simulink library "GearSystems"  (R2023b)
settings: Solver=VariableStepAuto  StartTime=0.0  StopTime=10.0  RelTol=1e-3
undefined symbols (not defined in the file or in its folder): manual_gearbox
settings Model: Creator=dadikozyanaa  LastModifiedBy=koenjacobs
settings DebuggingCC: UnconnectedInputMsg=warning  UnconnectedOutputMsg=warning  UnconnectedLineMsg=warning
settings ModelReferenceCC: EnableRefExpFcnMdlSchedulingChecks=on
settings RTWCC: DLArmComputeVersion=19.05

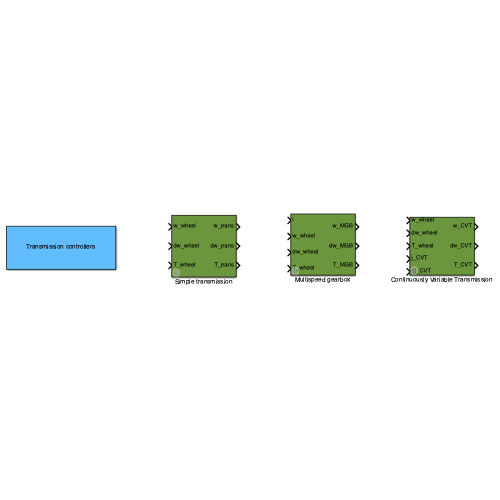
[thumbnail: Simulink's stored preview of the top-level diagram]
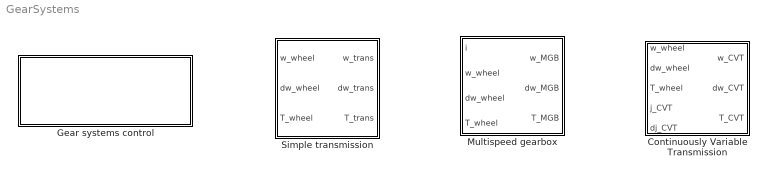
== system GearSystems ==
  Continuously Variable Transmission : Subsystem  Tag=cvt  mask(CVT){e_CVT=0.96, w_max=100, w_wheel_min=1}
      mask prompts: e_CVT "Efficiency [-]"; w_max "Maximum engine speed [rad/s]"; w_wheel_min "Minimum wheel speed beyond which losses are generated [rad/s]"
      mask help:
      | This block simulates a CVT transmission.
      |
      | Input:
      | =====
      | 	w_wheel	Speed of the wheel [rad/s]
      | 	dw_wheel	Acceleration of the wheel [rad/s^2],
      | 	T_wheel	Torque on the wheel [Nm]
      | 	j_CVT	Gear ratio [-]
      | 	dj_CVT	Change of gear ratio [1/s]
      |
      | Output:
      | ======
      | 	w_CVT	Speed of the fly wheel [rad/s]
      | 	dw_CVT	Acceleration of the fly wheel [rad/s^2]
      | 	T_CVT	Torque on the fly wheel [Nm]
      mask init:
      | init_CVT;
  Gear systems control : Subsystem
      settings: OpenFcn=GearSystemsControl
      mask Display:
      | disp(['Transmission controllers' ...
      |     ''])
  Multispeed gearbox : Subsystem  Tag=transmission  mask(Manual Gear Box){nr_gears=2, i_1=15.174, i_2=8.338, i_3=5.378, i_4=3.937, i_5=2.748, i_6=2.748, i_diff=1, e_GT=0.98, P_GT0=300, w_wheel_min=1}
      mask prompts: nr_gears "Select number of gears:"; i_1 "1. gear [-]"; i_2 "2. gear [-]"; i_3 "3. gear [-]"; i_4 "4. gear [-]"; i_5 "5. gear [-]"; i_6 "6. gear [-]"; i_diff "Differential gear [-]"; e_GT "Efficiency [-]"; P_GT0 "Idling losses (friction) [W]"; w_wheel_min "Minimum wheel speed beyond which losses are generated [rad/s]"
      mask help:
      | This block simulates a manual gear box.
      |
      | Input:
      | =====
      | 	w_wheel	Speed of the wheel [rad/s]
      | 	dw_wheel	Acceleration of the wheel [rad/s^2],
      | 	T_wheel	Torque on the wheel [Nm]
      | 	i	Gear number [-]
      |
      | Output:
      | ======
      | 	w_MGB	Speed of the fly wheel [rad/s]
      | 	dw_MGB	Acceleration of the fly wheel [rad/s^2]
      | 	T_MGB	Torque on the fly wheel [Nm]
      mask init:
      | init_MGB;
      | init_MGB_control;
      mask Help: Contact a.a.dadikozyan@student.tue.nl for help.
      mask TypeOptions nr_gears: 2 | 3 | 4 | 5 | 6
      mask Callback nr_gears:
      | maskStr = get_param(gcb,'nr_gears');
      | 
      | switch maskStr
      |     case '2'
      |         set_param(gcb,'MaskVisibilities',{'on';'on';'on';'off';'off';'off';'off';'on';'on';'on';'on'}),
      |     case '3'
      |         set_param(gcb,'MaskVisibilities',{'on';'on';'on';'on';'off';'off';'off';'on';'on';'on';'on'}),
      |     case '4'
      |         set_param(gcb,'MaskVisibilities',{'on';'on';'on';'on';'on';'off';'off';'on';'on';'on';'on'}),
      |     case '5'
      |         set_param(gcb,'MaskVisibilities',{'on';'on';'on';'on';'on';'on';'off';'on';'on';'on';'on'}),
      |     case '6'
      |         set_param(gcb,'MaskVisibilities',{'on';'on';'on';'on';'on';'on';'on';'on';'on';'on';'on'}),
      | end
      | 
      | %set_param(gcb,'editvalue',maskStr);
  Simple transmission : Subsystem  mask(Simple Transmission){gear_ratio=3, e_GT=0.98, P_GT0=50, w_wheel_min=1}
      mask prompts: gear_ratio "Gear ratio [-]"; e_GT "Efficiency [-]"; P_GT0 "Idling losses (friction) [W]"; w_wheel_min "Minimum wheel speed beyond which losses are generated [rad/s]"
      mask help:
      | This block simulates a transmission with a fixed gear ratio.
      |
      | Input:
      | =====
      | 	w_wheel	Speed of the wheel [rad/s]
      | 	dw_wheel	Acceleration of the wheel [rad/s^2]
      | 	T_wheel	Torque on the wheel [Nm]
      |
      | Output:
      | ======
      | 	w_trans	Speed of the fly wheel [rad/s]
      | 	dw_trans	Acceleration of the fly wheel [rad/s^2]
      | 	T_trans	Torque on the fly wheel [Nm]
      mask init:
      | init_transmission

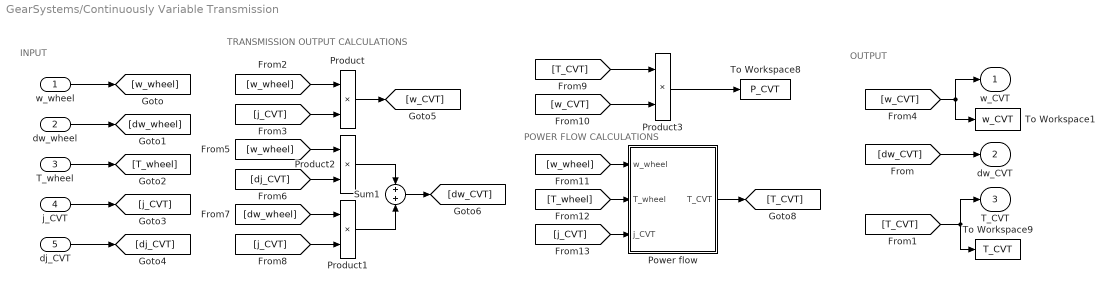
== system GearSystems/Continuously Variable Transmission ==
  note: POWER FLOW CALCULATIONS
  note: TRANSMISSION OUTPUT CALCULATIONS
  note: OUTPUT
  note: INPUT
  w_wheel : Inport
  dw_wheel : Inport  Port=2
  T_wheel : Inport  Port=3
  j_CVT : Inport  Port=4
  dj_CVT : Inport  Port=5
  Power flow : Subsystem
  Product{,1..3} (4 alike) : Product  InputSameDT=on  RndMeth=Zero  SaturateOnIntegerOverflow=on  OutDataTypeStr=Inherit: Same as first input
  Sum1 : Sum  Inputs=+|+
  To Workspace1 : ToWorkspace  VariableName=w_CVT  SampleTime=-1
  To Workspace8 : ToWorkspace  VariableName=P_CVT  SampleTime=-1
  To Workspace9 : ToWorkspace  VariableName=T_CVT  SampleTime=-1
  w_CVT : Outport  InitialOutput=0
  dw_CVT : Outport  Port=2  InitialOutput=0
  T_CVT : Outport  Port=3  InitialOutput=0
  wires:
  Product1/1 -> Sum1/2
  Product2/1 -> Sum1/1
  w_wheel/1 -> [w_wheel]
  dw_wheel/1 -> [dw_wheel]
  T_wheel/1 -> [T_wheel]
  j_CVT/1 -> [j_CVT]
  dj_CVT/1 -> [dj_CVT]
  [j_CVT] -> Product/2
  [w_wheel] -> Product/1
  [w_wheel] -> Product2/1
  [j_CVT] -> Product1/2
  [dj_CVT] -> Product2/2
  [dw_wheel] -> Product1/1
  Product/1 -> [w_CVT]
  Sum1/1 -> [dw_CVT]
  [w_CVT] -> Product3/2
  [T_CVT] -> Product3/1
  Product3/1 -> To Workspace8/1
  Power flow/1(T_CVT) -> [T_CVT]
  [w_wheel] -> Power flow/1(w_wheel)
  [T_wheel] -> Power flow/2(T_wheel)
  [j_CVT] -> Power flow/3(j_CVT)
  [w_CVT] -> To Workspace1/1, w_CVT/1
  [dw_CVT] -> dw_CVT/1
  [T_CVT] -> To Workspace9/1, T_CVT/1

== system GearSystems/Gear systems control ==

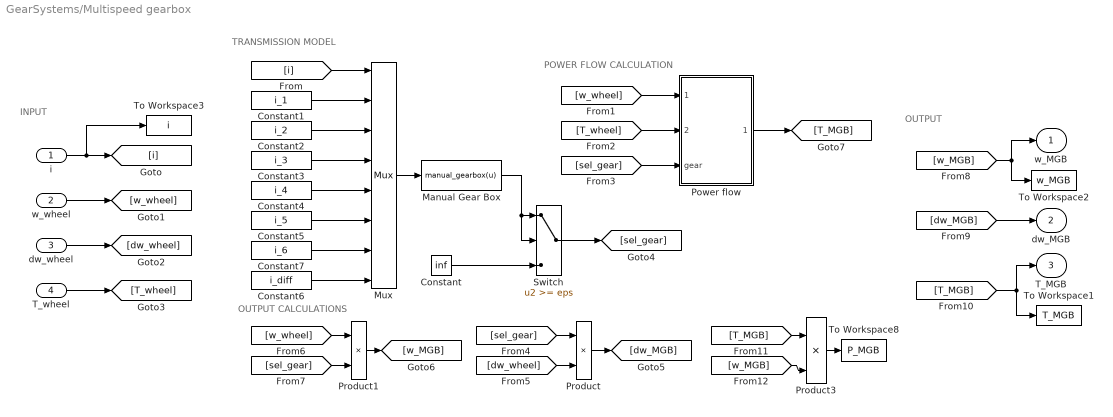
== system GearSystems/Multispeed gearbox ==
  note: OUTPUT CALCULATIONS
  note: POWER FLOW CALCULATION
  note: TRANSMISSION MODEL
  note: OUTPUT
  note: INPUT
  i : Inport
  w_wheel : Inport  Port=2
  dw_wheel : Inport  Port=3
  T_wheel : Inport  Port=4
  Constant : Constant  Value=inf
  Constant1 : Constant  Value=i_1
  Constant2 : Constant  Value=i_2
  Constant3 : Constant  Value=i_3
  Constant4 : Constant  Value=i_4
  Constant5 : Constant  Value=i_5
  Constant6 : Constant  Value=i_diff
  Constant7 : Constant  Value=i_6
  Manual Gear Box : MATLABFcn  MATLABFcn=manual_gearbox(u)  OutputDimensions=1
      mask Display: disp('Gear selection');
  Mux : Mux  Inputs=8
  Power flow : Subsystem
  Product : Product  InputSameDT=on  RndMeth=Zero  SaturateOnIntegerOverflow=on  OutDataTypeStr=Inherit: Same as first input
  Product1 : Product  InputSameDT=on  RndMeth=Zero  SaturateOnIntegerOverflow=on  OutDataTypeStr=Inherit: Same as first input
  Product3 : Product  InputSameDT=on  RndMeth=Zero  SaturateOnIntegerOverflow=on  OutDataTypeStr=Inherit: Same as first input
  Switch : Switch  Threshold=eps
  To Workspace1 : ToWorkspace  VariableName=T_MGB  SampleTime=-1
  To Workspace2 : ToWorkspace  VariableName=w_MGB  SampleTime=-1
  To Workspace3 : ToWorkspace  VariableName=i  SampleTime=-1
  To Workspace8 : ToWorkspace  VariableName=P_MGB  SampleTime=-1
  w_MGB : Outport  InitialOutput=0
  dw_MGB : Outport  Port=2  InitialOutput=0
  T_MGB : Outport  Port=3  InitialOutput=0
  wires:
  Constant/1 -> Switch/3
  Constant1/1 -> Mux/2
  Constant2/1 -> Mux/3
  Constant3/1 -> Mux/4
  Constant4/1 -> Mux/5
  Constant5/1 -> Mux/6
  Constant6/1 -> Mux/8
  Constant7/1 -> Mux/7
  w_wheel/1 -> [w_wheel]
  i/1 -> To Workspace3/1, [i]
  dw_wheel/1 -> [dw_wheel]
  T_wheel/1 -> [T_wheel]
  [i] -> Mux/1
  Mux/1 -> Manual Gear Box/1
  Manual Gear Box/1 -> Switch/2, Switch/1
  Switch/1 -> [sel_gear]
  [sel_gear] -> Product/1
  [dw_wheel] -> Product/2
  [w_wheel] -> Product1/1
  [sel_gear] -> Product1/2
  Product/1 -> [dw_MGB]
  Product1/1 -> [w_MGB]
  [w_MGB] -> To Workspace2/1, w_MGB/1
  [dw_MGB] -> dw_MGB/1
  [T_MGB] -> To Workspace1/1, T_MGB/1
  Product3/1 -> To Workspace8/1
  [T_MGB] -> Product3/1
  [w_MGB] -> Product3/2
  Power flow/1(T_MGB) -> [T_MGB]
  [T_wheel] -> Power flow/2(T_wheel)
  [w_wheel] -> Power flow/1(w_wheel)
  [sel_gear] -> Power flow/3(gear)

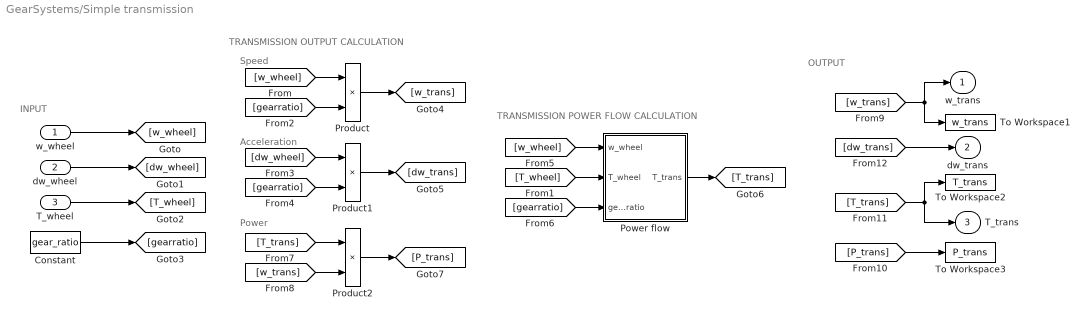
== system GearSystems/Simple transmission ==
  note: OUTPUT
  note: Speed
  note: TRANSMISSION POWER FLOW CALCULATION
  note: TRANSMISSION OUTPUT CALCULATION
  note: INPUT
  note: Acceleration
  note: Power
  w_wheel : Inport
  dw_wheel : Inport  Port=2
  T_wheel : Inport  Port=3
  Constant : Constant  Value=gear_ratio
  Power flow : Subsystem
  Product : Product  InputSameDT=on  RndMeth=Zero  SaturateOnIntegerOverflow=on  OutDataTypeStr=Inherit: Same as first input
  Product1 : Product  InputSameDT=on  RndMeth=Zero  SaturateOnIntegerOverflow=on  OutDataTypeStr=Inherit: Same as first input
  Product2 : Product  InputSameDT=on  RndMeth=Zero  SaturateOnIntegerOverflow=on  OutDataTypeStr=Inherit: Same as first input
  To Workspace1 : ToWorkspace  VariableName=w_trans  SampleTime=-1
  To Workspace2 : ToWorkspace  VariableName=T_trans  SampleTime=-1
  To Workspace3 : ToWorkspace  VariableName=P_trans  SampleTime=-1
  w_trans : Outport  InitialOutput=0
  dw_trans : Outport  Port=2  InitialOutput=0
  T_trans : Outport  Port=3  InitialOutput=0
  wires:
  T_wheel/1 -> [T_wheel]
  dw_wheel/1 -> [dw_wheel]
  w_wheel/1 -> [w_wheel]
  Constant/1 -> [gearratio]
  [w_wheel] -> Product/1
  [gearratio] -> Product/2
  [dw_wheel] -> Product1/1
  [gearratio] -> Product1/2
  Product1/1 -> [dw_trans]
  Power flow/1(T_trans) -> [T_trans]
  [w_wheel] -> Power flow/1(w_wheel)
  [T_wheel] -> Power flow/2(T_wheel)
  [gearratio] -> Power flow/3(gear_ratio)
  [T_trans] -> Product2/1
  [w_trans] -> Product2/2
  Product2/1 -> [P_trans]
  Product/1 -> [w_trans]
  [w_trans] -> To Workspace1/1, w_trans/1
  [P_trans] -> To Workspace3/1
  [T_trans] -> To Workspace2/1, T_trans/1
  [dw_trans] -> dw_trans/1

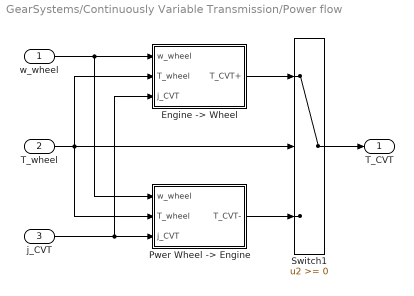
== system GearSystems/Continuously Variable Transmission/Power flow ==
  w_wheel : Inport
  T_wheel : Inport  Port=2
  j_CVT : Inport  Port=3
  "Engine -> Wheel" : Subsystem
  "Pwer Wheel -> Engine" : Subsystem
  Switch1 : Switch
  T_CVT : Outport  InitialOutput=0
  wires:
  "Pwer Wheel -> Engine"/1(T_CVT-) -> Switch1/3
  "Engine -> Wheel"/1(T_CVT+) -> Switch1/1
  Switch1/1 -> T_CVT/1
  j_CVT/1 -> "Engine -> Wheel"/3(j_CVT), "Pwer Wheel -> Engine"/3(j_CVT)
  w_wheel/1 -> "Pwer Wheel -> Engine"/1(w_wheel), "Engine -> Wheel"/1(w_wheel)
  T_wheel/1 -> "Pwer Wheel -> Engine"/2(T_wheel), "Engine -> Wheel"/2(T_wheel), Switch1/2

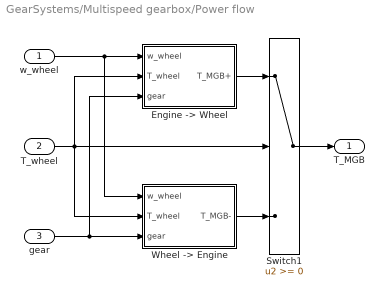
== system GearSystems/Multispeed gearbox/Power flow ==
  w_wheel : Inport
  T_wheel : Inport  Port=2
  gear : Inport  Port=3
  "Engine -> Wheel" : Subsystem
  Switch1 : Switch
  "Wheel -> Engine" : Subsystem
  T_MGB : Outport  InitialOutput=0
  wires:
  w_wheel/1 -> "Wheel -> Engine"/1(w_wheel), "Engine -> Wheel"/1(w_wheel)
  gear/1 -> "Wheel -> Engine"/3(gear), "Engine -> Wheel"/3(gear)
  "Wheel -> Engine"/1(T_MGB-) -> Switch1/3
  T_wheel/1 -> "Wheel -> Engine"/2(T_wheel), "Engine -> Wheel"/2(T_wheel), Switch1/2
  "Engine -> Wheel"/1(T_MGB+) -> Switch1/1
  Switch1/1 -> T_MGB/1

== system GearSystems/Simple transmission/Power flow ==
  w_wheel : Inport
  T_wheel : Inport  Port=2
  gear_ratio : Inport  Port=3
  "Energy Engine -> Wheel" : Subsystem
  "Energy Wheel -> Engine" : Subsystem
  Switch1 : Switch
  T_trans : Outport  InitialOutput=0
  wires:
  gear_ratio/1 -> "Energy Wheel -> Engine"/3(gear_ratio), "Energy Engine -> Wheel"/3(gear_ratio)
  Switch1/1 -> T_trans/1
  "Energy Engine -> Wheel"/1(T_trans+) -> Switch1/1
  w_wheel/1 -> "Energy Wheel -> Engine"/1(w_wheel), "Energy Engine -> Wheel"/1(w_wheel)
  "Energy Wheel -> Engine"/1(T_trans-) -> Switch1/3
  T_wheel/1 -> "Energy Wheel -> Engine"/2(T_wheel), "Energy Engine -> Wheel"/2(T_wheel), Switch1/2

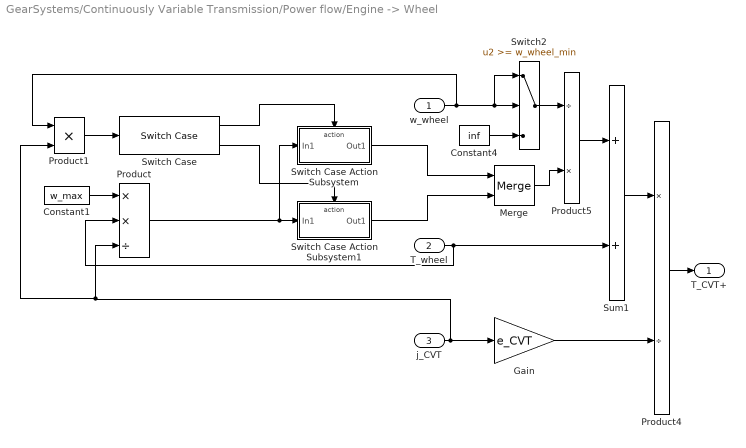
== system GearSystems/Continuously Variable Transmission/Power flow/Engine -> Wheel ==
  w_wheel : Inport
  T_wheel : Inport  Port=2
  j_CVT : Inport  Port=3
  Constant1 : Constant  Value=w_max
  Constant4 : Constant  Value=inf
  Gain : Gain  Gain=e_CVT  SaturateOnIntegerOverflow=on  OutDataTypeStr=Inherit: Same as input  ParamDataTypeStr=Inherit: Same as input
  Merge : Merge
  Product : Product  Inputs=**/
  Product1 : Product
  Product4 : Product  Inputs=*/  InputSameDT=on  RndMeth=Zero  SaturateOnIntegerOverflow=on  OutDataTypeStr=Inherit: Same as first input
  Product5 : Product  Inputs=/*  InputSameDT=on  RndMeth=Zero  SaturateOnIntegerOverflow=on  OutDataTypeStr=Inherit: Same as first input
  Sum1 : Sum  InputSameDT=on  SaturateOnIntegerOverflow=on  OutDataTypeStr=Inherit: Same as first input
  Switch Case : SwitchCase  CaseConditions={floor(0.5*w_max)}
  Switch Case Action Subsystem : Subsystem  TreatAsAtomicUnit=on
  Switch Case Action Subsystem1 : Subsystem  TreatAsAtomicUnit=on
  Switch2 : Switch  Threshold=w_wheel_min
  T_CVT+ : Outport  InitialOutput=0
  wires:
  Gain/1 -> Product4/2
  Product4/1 -> T_CVT+/1
  Sum1/1 -> Product4/1
  T_wheel/1 -> Product/2, Sum1/2
  Product5/1 -> Sum1/1
  w_wheel/1 -> Product1/1, Switch2/1, Switch2/2
  Constant4/1 -> Switch2/3
  Switch2/1 -> Product5/1
  Merge/1 -> Product5/2
  j_CVT/1 -> Product1/2, Product/3, Gain/1
  Switch Case Action Subsystem1/1(Out1) -> Merge/2
  Switch Case Action Subsystem/1(Out1) -> Merge/1
  Switch Case/1 -> Switch Case Action Subsystem/Action
  Switch Case/2 -> Switch Case Action Subsystem1/Action
  Product/1 -> Switch Case Action Subsystem1/1(In1), Switch Case Action Subsystem/1(In1)
  Constant1/1 -> Product/1
  Product1/1 -> Switch Case/1

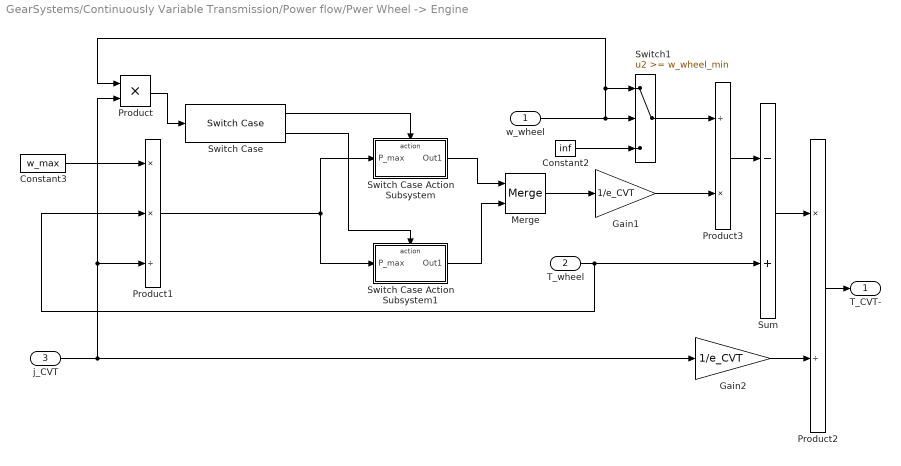
== system GearSystems/Continuously Variable Transmission/Power flow/Pwer Wheel -> Engine ==
  w_wheel : Inport
  T_wheel : Inport  Port=2
  j_CVT : Inport  Port=3
  Constant2 : Constant  Value=inf
  Constant3 : Constant  Value=w_max
  Gain1 : Gain  Gain=1/e_CVT  SaturateOnIntegerOverflow=on  OutDataTypeStr=Inherit: Same as input  ParamDataTypeStr=Inherit: Same as input
  Gain2 : Gain  Gain=1/e_CVT  SaturateOnIntegerOverflow=on  OutDataTypeStr=Inherit: Same as input  ParamDataTypeStr=Inherit: Same as input
  Merge : Merge
  Product : Product
  Product1 : Product  Inputs=**/  InputSameDT=on  RndMeth=Zero  SaturateOnIntegerOverflow=on  OutDataTypeStr=Inherit: Same as first input
  Product2 : Product  Inputs=*/  InputSameDT=on  RndMeth=Zero  SaturateOnIntegerOverflow=on  OutDataTypeStr=Inherit: Same as first input
  Product3 : Product  Inputs=/*  InputSameDT=on  RndMeth=Zero  SaturateOnIntegerOverflow=on  OutDataTypeStr=Inherit: Same as first input
  Sum : Sum  Inputs=-+  InputSameDT=on  SaturateOnIntegerOverflow=on  OutDataTypeStr=Inherit: Same as first input
  Switch Case : SwitchCase  CaseConditions={floor(0.5*w_max)}
  Switch Case Action Subsystem : Subsystem  TreatAsAtomicUnit=on
  Switch Case Action Subsystem1 : Subsystem  TreatAsAtomicUnit=on
  Switch1 : Switch  Threshold=w_wheel_min
  T_CVT- : Outport  InitialOutput=0
  wires:
  Sum/1 -> Product2/1
  Gain1/1 -> Product3/2
  Switch1/1 -> Product3/1
  Product3/1 -> Sum/1
  Product2/1 -> T_CVT-/1
  w_wheel/1 -> Switch1/1, Product/1, Switch1/2
  Merge/1 -> Gain1/1
  Constant2/1 -> Switch1/3
  Gain2/1 -> Product2/2
  T_wheel/1 -> Product1/2, Sum/2
  Product1/1 -> Switch Case Action Subsystem/1(P_max), Switch Case Action Subsystem1/1(P_max)
  j_CVT/1 -> Gain2/1, Product/2, Product1/3
  Constant3/1 -> Product1/1
  Switch Case/2 -> Switch Case Action Subsystem1/Action
  Switch Case Action Subsystem/1(Out1) -> Merge/1
  Switch Case Action Subsystem1/1(Out1) -> Merge/2
  Product/1 -> Switch Case/1
  Switch Case/1 -> Switch Case Action Subsystem/Action

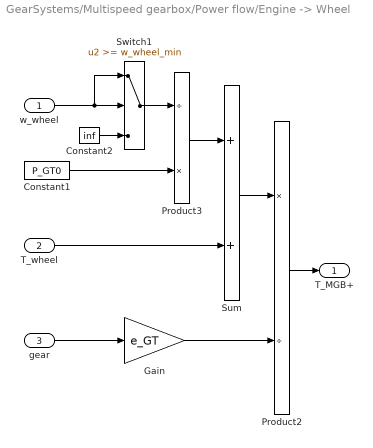
== system GearSystems/Multispeed gearbox/Power flow/Engine -> Wheel ==
  w_wheel : Inport
  T_wheel : Inport  Port=2
  gear : Inport  Port=3
  Constant1 : Constant  Value=P_GT0
  Constant2 : Constant  Value=inf
  Gain : Gain  Gain=e_GT  SaturateOnIntegerOverflow=on  OutDataTypeStr=Inherit: Same as input  ParamDataTypeStr=Inherit: Same as input
  Product2 : Product  Inputs=*/  InputSameDT=on  RndMeth=Zero  SaturateOnIntegerOverflow=on  OutDataTypeStr=Inherit: Same as first input
  Product3 : Product  Inputs=/*  InputSameDT=on  RndMeth=Zero  SaturateOnIntegerOverflow=on  OutDataTypeStr=Inherit: Same as first input
  Sum : Sum  InputSameDT=on  SaturateOnIntegerOverflow=on  OutDataTypeStr=Inherit: Same as first input
  Switch1 : Switch  Threshold=w_wheel_min
  T_MGB+ : Outport  InitialOutput=0
  wires:
  T_wheel/1 -> Sum/2
  Product3/1 -> Sum/1
  Gain/1 -> Product2/2
  Product2/1 -> T_MGB+/1
  Sum/1 -> Product2/1
  w_wheel/1 -> Switch1/2, Switch1/1
  Constant2/1 -> Switch1/3
  Switch1/1 -> Product3/1
  Constant1/1 -> Product3/2
  gear/1 -> Gain/1

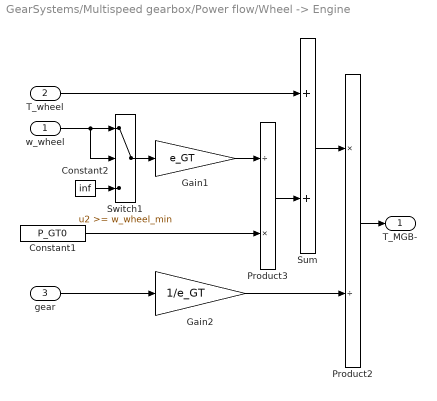
== system GearSystems/Multispeed gearbox/Power flow/Wheel -> Engine ==
  w_wheel : Inport
  T_wheel : Inport  Port=2
  gear : Inport  Port=3
  Constant1 : Constant  Value=P_GT0
  Constant2 : Constant  Value=inf
  Gain1 : Gain  Gain=e_GT  SaturateOnIntegerOverflow=on  OutDataTypeStr=Inherit: Same as input  ParamDataTypeStr=Inherit: Same as input
  Gain2 : Gain  Gain=1/e_GT  SaturateOnIntegerOverflow=on  OutDataTypeStr=Inherit: Same as input  ParamDataTypeStr=Inherit: Same as input
  Product2 : Product  Inputs=*/  InputSameDT=on  RndMeth=Zero  SaturateOnIntegerOverflow=on  OutDataTypeStr=Inherit: Same as first input
  Product3 : Product  Inputs=/*  InputSameDT=on  RndMeth=Zero  SaturateOnIntegerOverflow=on  OutDataTypeStr=Inherit: Same as first input
  Sum : Sum  InputSameDT=on  SaturateOnIntegerOverflow=on  OutDataTypeStr=Inherit: Same as first input
  Switch1 : Switch  Threshold=w_wheel_min
  T_MGB- : Outport  InitialOutput=0
  wires:
  w_wheel/1 -> Switch1/1, Switch1/2
  gear/1 -> Gain2/1
  Constant2/1 -> Switch1/3
  Switch1/1 -> Gain1/1
  Constant1/1 -> Product3/2
  T_wheel/1 -> Sum/1
  Gain2/1 -> Product2/2
  Product2/1 -> T_MGB-/1
  Product3/1 -> Sum/2
  Sum/1 -> Product2/1
  Gain1/1 -> Product3/1

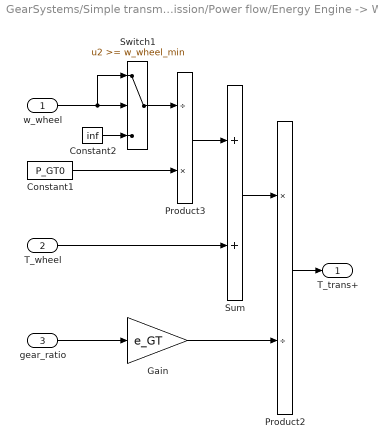
== system GearSystems/Simple transmission/Power flow/Energy Engine -> Wheel ==
  w_wheel : Inport
  T_wheel : Inport  Port=2
  gear_ratio : Inport  Port=3
  Constant1 : Constant  Value=P_GT0
  Constant2 : Constant  Value=inf
  Gain : Gain  Gain=e_GT  SaturateOnIntegerOverflow=on  OutDataTypeStr=Inherit: Same as input  ParamDataTypeStr=Inherit: Same as input
  Product2 : Product  Inputs=*/  InputSameDT=on  RndMeth=Zero  SaturateOnIntegerOverflow=on  OutDataTypeStr=Inherit: Same as first input
  Product3 : Product  Inputs=/*  InputSameDT=on  RndMeth=Zero  SaturateOnIntegerOverflow=on  OutDataTypeStr=Inherit: Same as first input
  Sum : Sum  InputSameDT=on  SaturateOnIntegerOverflow=on  OutDataTypeStr=Inherit: Same as first input
  Switch1 : Switch  Threshold=w_wheel_min
  T_trans+ : Outport  InitialOutput=0
  wires:
  Product2/1 -> T_trans+/1
  w_wheel/1 -> Switch1/2, Switch1/1
  Sum/1 -> Product2/1
  Constant1/1 -> Product3/2
  Product3/1 -> Sum/1
  Switch1/1 -> Product3/1
  Gain/1 -> Product2/2
  Constant2/1 -> Switch1/3
  T_wheel/1 -> Sum/2
  gear_ratio/1 -> Gain/1

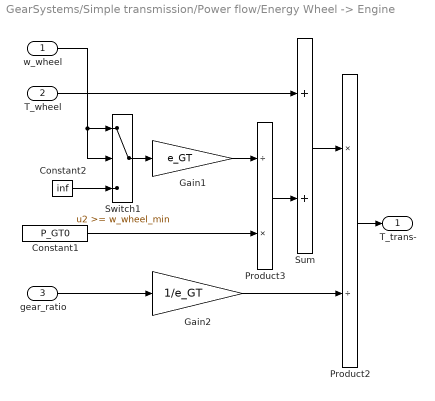
== system GearSystems/Simple transmission/Power flow/Energy Wheel -> Engine ==
  w_wheel : Inport
  T_wheel : Inport  Port=2
  gear_ratio : Inport  Port=3
  Constant1 : Constant  Value=P_GT0
  Constant2 : Constant  Value=inf
  Gain1 : Gain  Gain=e_GT  SaturateOnIntegerOverflow=on  OutDataTypeStr=Inherit: Same as input  ParamDataTypeStr=Inherit: Same as input
  Gain2 : Gain  Gain=1/e_GT  SaturateOnIntegerOverflow=on  OutDataTypeStr=Inherit: Same as input  ParamDataTypeStr=Inherit: Same as input
  Product2 : Product  Inputs=*/  InputSameDT=on  RndMeth=Zero  SaturateOnIntegerOverflow=on  OutDataTypeStr=Inherit: Same as first input
  Product3 : Product  Inputs=/*  InputSameDT=on  RndMeth=Zero  SaturateOnIntegerOverflow=on  OutDataTypeStr=Inherit: Same as first input
  Sum : Sum  InputSameDT=on  SaturateOnIntegerOverflow=on  OutDataTypeStr=Inherit: Same as first input
  Switch1 : Switch  Threshold=w_wheel_min
  T_trans- : Outport  InitialOutput=0
  wires:
  T_wheel/1 -> Sum/1
  Constant1/1 -> Product3/2
  gear_ratio/1 -> Gain2/1
  w_wheel/1 -> Switch1/1, Switch1/2
  Gain2/1 -> Product2/2
  Switch1/1 -> Gain1/1
  Product2/1 -> T_trans-/1
  Product3/1 -> Sum/2
  Constant2/1 -> Switch1/3
  Sum/1 -> Product2/1
  Gain1/1 -> Product3/1

== system GearSystems/Continuously Variable Transmission/Power flow/Engine -> Wheel/Switch Case Action Subsystem ==
  In1 : Inport
  Action Port : ActionPort
  Gain : Gain  Gain=0.06
  Out1 : Outport
  wires:
  In1/1 -> Gain/1
  Gain/1 -> Out1/1

== system GearSystems/Continuously Variable Transmission/Power flow/Engine -> Wheel/Switch Case Action Subsystem1 ==
  In1 : Inport
  Action Port : ActionPort
  Gain : Gain  Gain=0.04
  Out1 : Outport
  wires:
  In1/1 -> Gain/1
  Gain/1 -> Out1/1

== system GearSystems/Continuously Variable Transmission/Power flow/Pwer Wheel -> Engine/Switch Case Action Subsystem ==
  P_max : Inport
  Action Port : ActionPort  ActionPortLabel=case [ 50 ]:
  Gain : Gain  Gain=0.06
  Out1 : Outport
  wires:
  P_max/1 -> Gain/1
  Gain/1 -> Out1/1

== system GearSystems/Continuously Variable Transmission/Power flow/Pwer Wheel -> Engine/Switch Case Action Subsystem1 ==
  P_max : Inport
  Action Port : ActionPort
  Gain : Gain  Gain=0.04
  Out1 : Outport
  wires:
  P_max/1 -> Gain/1
  Gain/1 -> Out1/1
